simulink model "Tuto5"  (R2018b)
settings: Solver=VariableStepAuto  StartTime=0.0  StopTime=10.0  RelTol=1e-3
libraries: fl_lib x12, nesl_utility x6
settings Model: Creator=77498  LastModifiedBy=77498

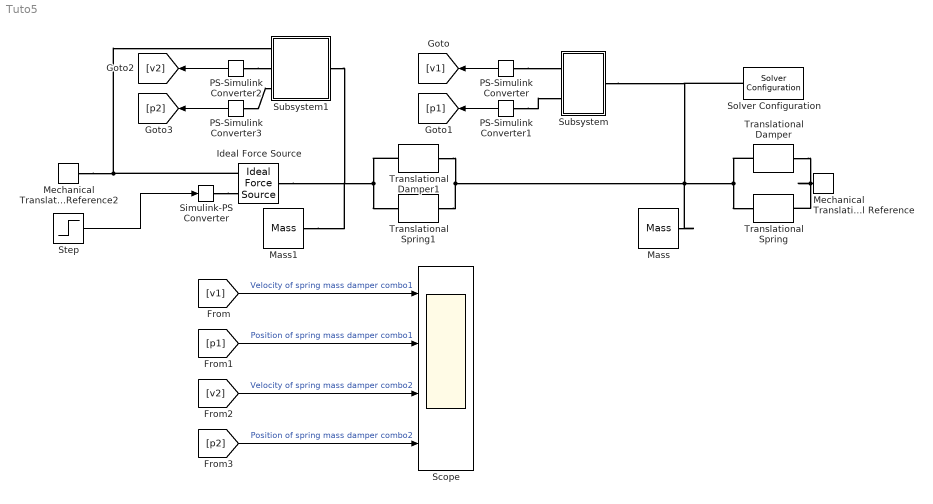
== system Tuto5 ==
  Ideal Force Source : fl_lib/Mechanical/Mechanical Sources/Ideal Force Source
  Mass : fl_lib/Mechanical/Translational Elements/Mass  mass=1 kg  v_specify=off  v_priority=High  v=0 m/s  v_nominal_specify=off  v_nominal_unit=m/s  v_nominal_value=1  f_specify=off  f_priority=None  f=0 N  f_nominal_specify=off  f_nominal_unit=N  f_nominal_value=1
  Mass1 : fl_lib/Mechanical/Translational Elements/Mass  mass=1 kg  v_specify=off  v_priority=High  v=0 m/s  v_nominal_specify=off  v_nominal_unit=m/s  v_nominal_value=1  f_specify=off  f_priority=None  f=0 N  f_nominal_specify=off  f_nominal_unit=N  f_nominal_value=1
  Mechanical Translational Reference : fl_lib/Mechanical/Translational Elements/Mechanical Translational Reference
  Mechanical Translational Reference2 : fl_lib/Mechanical/Translational Elements/Mechanical Translational Reference
  PS-Simulink Converter : nesl_utility/PS-Simulink Converter  PhysicalDomain=network_engine_domain  SubClassName=ps_output  LeftPortType=input  RightPortType=output  PseudoPeriodic=off  Frequencies=[]  Unit=m/s  AffineConversion=off
  PS-Simulink Converter1 : nesl_utility/PS-Simulink Converter  PhysicalDomain=network_engine_domain  SubClassName=ps_output  LeftPortType=input  RightPortType=output  PseudoPeriodic=off  Frequencies=[]  Unit=m  AffineConversion=off
  PS-Simulink Converter2 : nesl_utility/PS-Simulink Converter  PhysicalDomain=network_engine_domain  SubClassName=ps_output  LeftPortType=input  RightPortType=output  PseudoPeriodic=off  Frequencies=[]  Unit=m/s  AffineConversion=off
  PS-Simulink Converter3 : nesl_utility/PS-Simulink Converter  PhysicalDomain=network_engine_domain  SubClassName=ps_output  LeftPortType=input  RightPortType=output  PseudoPeriodic=off  Frequencies=[]  Unit=m  AffineConversion=off
  Scope : Scope  NumInputPorts=4
  Simulink-PS Converter : nesl_utility/Simulink-PS Converter  PhysicalDomain=network_engine_domain  SubClassName=ps_input  LeftPortType=input  RightPortType=output  PseudoPeriodic=off  Frequencies=[]  NoiseDistribution=none  NoiseParameters=[]  Unit=N  AffineConversion=off  FilteringAndDerivatives=provide  SimscapeFilterOrder=1  InputFilterTimeConstant=0.001  UdotUserProvided=0
  Solver Configuration : nesl_utility/Solver Configuration  PhysicalDomain=network_engine_domain  SubClassName=solver  LeftPortType=input  RightPortType=generic  Tones=[]  Harmonics=[]  SimulateNoise=off  Profile=off  UseLocalSampling=off  EnableSwitchedLinearOptims=on  FrequencyDomain=off  UseCCode=off  RelTol=0.001  AbsTol=1e-06  MinStep=1e-09  ToWorkspace=off  RevertToSquareIcSolve=off  NumHomotopyIterations=100  PhasorMode=off  PhasorModeNumHarmonics=1  DoDC=off  ResidualTolerance=1e-09  UseLocalSolver=off  LocalSolverChoice=NE_BACKWARD_EULER_ADVANCER  LocalSolverSampleTime=0.001  DoFixedCost=off  MaxNonlinIter=3  MaxModeIter=2  LinearAlgebra=auto  EquationFormulation=NE_TIME_EF  DelaysMemoryBudget=1024  AutomaticFiltering=on  FilteringTimeConstant=0.001  PartitionStorageMethod=AS_NEEDED  PartitionMemoryBudget=1024
  Step : Step  After=500  SampleTime=0
  Subsystem : Subsystem
  Subsystem1 : Subsystem
  Translational Damper : fl_lib/Mechanical/Translational Elements/Translational Damper  D=5 N/(m/s)  v_specify=off  v_priority=None  v=0 m/s  v_nominal_specify=off  v_nominal_unit=m/s  v_nominal_value=1  f_specify=off  f_priority=None  f=0 N  f_nominal_specify=off  f_nominal_unit=N  f_nominal_value=1
  Translational Damper1 : fl_lib/Mechanical/Translational Elements/Translational Damper  D=5 N/(m/s)  v_specify=off  v_priority=None  v=0 m/s  v_nominal_specify=off  v_nominal_unit=m/s  v_nominal_value=1  f_specify=off  f_priority=None  f=0 N  f_nominal_specify=off  f_nominal_unit=N  f_nominal_value=1
  Translational Spring : fl_lib/Mechanical/Translational Elements/Translational Spring  spr_rate=400 N/m  v_specify=off  v_priority=None  v=0 m/s  v_nominal_specify=off  v_nominal_unit=m/s  v_nominal_value=1  f_specify=off  f_priority=None  f=0 N  f_nominal_specify=off  f_nominal_unit=N  f_nominal_value=1  x_specify=off  x_priority=High  x=0 m  x_nominal_specify=off  x_nominal_unit=m  x_nominal_value=1
  Translational Spring1 : fl_lib/Mechanical/Translational Elements/Translational Spring  spr_rate=400 N/m  v_specify=off  v_priority=None  v=0 m/s  v_nominal_specify=off  v_nominal_unit=m/s  v_nominal_value=1  f_specify=off  f_priority=None  f=0 N  f_nominal_specify=off  f_nominal_unit=N  f_nominal_value=1  x_specify=off  x_priority=High  x=0 m  x_nominal_specify=off  x_nominal_unit=m  x_nominal_value=1
  wires:
  Step/1 -> Simulink-PS Converter/1
  PS-Simulink Converter/1 -> [v1]
  PS-Simulink Converter1/1 -> [p1]
  PS-Simulink Converter2/1 -> [v2]
  PS-Simulink Converter3/1 -> [p2]
  [v2] -> Scope/3  "Velocity of spring mass damper combo2"
  [p1] -> Scope/2  "Position of spring mass damper combo1"
  [v1] -> Scope/1  "Velocity of spring mass damper combo1"
  [p2] -> Scope/4  "Position of spring mass damper combo2"
  connections:
  Translational Damper/RConn1 -- Translational Spring/RConn1 -- Mechanical Translational Reference/LConn1
  Translational Damper1/RConn1 -- Translational Spring1/RConn1 -- Solver Configuration/RConn1 -- Subsystem/LConn1 -- Mass/LConn1 -- Translational Damper/LConn1 -- Translational Spring/LConn1
  Translational Damper1/LConn1 -- Subsystem1/LConn1 -- Mass1/LConn1 -- Ideal Force Source/LConn1 -- Translational Spring1/LConn1
  Mechanical Translational Reference2/LConn1 -- Subsystem1/RConn1 -- Ideal Force Source/RConn2
  Simulink-PS Converter/RConn1 -- Ideal Force Source/RConn1
  PS-Simulink Converter/LConn1 -- Subsystem/RConn1
  PS-Simulink Converter1/LConn1 -- Subsystem/RConn2
  PS-Simulink Converter2/LConn1 -- Subsystem1/RConn2
  PS-Simulink Converter3/LConn1 -- Subsystem1/RConn3

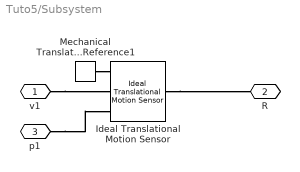
== system Tuto5/Subsystem ==
  Ideal Translational Motion Sensor : fl_lib/Mechanical/Mechanical Sensors/Ideal Translational Motion Sensor  offset=0 m
  Mechanical Translational Reference1 : fl_lib/Mechanical/Translational Elements/Mechanical Translational Reference
  v1 : PMIOPort  Side=Right
  R : PMIOPort  Port=2  Side=Left
  p1 : PMIOPort  Port=3  Side=Right
  connections:
  Mechanical Translational Reference1/LConn1 -- Ideal Translational Motion Sensor/RConn1
  v1/RConn1 -- Ideal Translational Motion Sensor/RConn2
  Ideal Translational Motion Sensor/LConn1 -- R/RConn1
  p1/RConn1 -- Ideal Translational Motion Sensor/RConn3

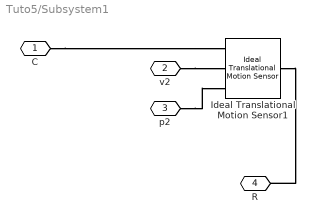
== system Tuto5/Subsystem1 ==
  Ideal Translational Motion Sensor1 : fl_lib/Mechanical/Mechanical Sensors/Ideal Translational Motion Sensor  offset=0 m
  C : PMIOPort  Side=Right
  v2 : PMIOPort  Port=2  Side=Right
  p2 : PMIOPort  Port=3  Side=Right
  R : PMIOPort  Port=4  Side=Left
  connections:
  Ideal Translational Motion Sensor1/LConn1 -- R/RConn1
  C/RConn1 -- Ideal Translational Motion Sensor1/RConn1
  v2/RConn1 -- Ideal Translational Motion Sensor1/RConn2
  p2/RConn1 -- Ideal Translational Motion Sensor1/RConn3
